simulink model "IEEE123bus_v2019b_Phasor_DPL"  (R2019b)
(part 2 of 7)

  86 : powerlib/Measurements/Three-Phase V-I Measurement  VoltageMeasurement=phase-to-ground  SetLabelV=on  LabelV=V86  Vpu=off  VpuLL=off  CurrentMeasurement=no  SetLabelI=on  LabelI=I65  Ipu=off  Pbase=100e6  Vbase=24900  OutputType=Complex  PhasorSimulation=on  PSBequivalent=0
      settings: SourceProductName=Simscape Electrical
  86 Y PQ : powerlib/Elements/Series RLC Load  LConnTagsString=a  RConnTagsString=__new0  NominalVoltage=1.0*2401.78  NominalFrequency=60  ActivePower=20e3*a  InductivePower=10e3*a  CapacitivePower=0  Setx0=off  InitialVoltage=0  SetiL0=off  InitialCurrent=0  Measurements=None  LoadType=constant PQ
      settings: SourceProductName=Simscape Electrical
  86-87 6 : powerlib/Elements/Distributed Parameters Line  Phases=3  Frequency=60  Resistance=R_3  Inductance=L_3  Capacitance=C_3  Length=450*ft2km  x1=[389.725132711134 3943.58441849278 4019.51592014074;376.991118430775 376.991118430775 376.991118430775;-0.630315628678231 0.166490215186273 1.73524344028808]  x2=[385.27258123151 3942.93848605317 4018.29081213384;376.991118430775 376.991118430775 376.991118430775;-0.627315579650631 0.165297691929816 1.73478902283365]  x3=[26.3237616446647 61.837520404268 25.7980203244257;376.991118430775 376.991118430775 376.991118430775;1.04881280773098 -2.64926297577553 -1.54351880159372]  x4=[26.4518860227079 84.1852813616711 55.6703006140533;376.991118430775 376.991118430775 376.991118430775;-2.0544828369136 0.403647758672959 1.6716643848458]  x5=5.64367487766549e-07  V1=ones(3,3)  V2=ones(3,3)  I1=ones(3,3)  I2=ones(3,3)  nHarmo=1  Measurements=None
      settings: SourceProductName=Simscape Electrical
  87 : powerlib/Measurements/Three-Phase V-I Measurement  VoltageMeasurement=phase-to-ground  SetLabelV=on  LabelV=V87  Vpu=off  VpuLL=off  CurrentMeasurement=no  SetLabelI=on  LabelI=I65  Ipu=off  Pbase=100e6  Vbase=24900  OutputType=Complex  PhasorSimulation=on  PSBequivalent=0
      settings: SourceProductName=Simscape Electrical
  87 Y PQ : powerlib/Elements/Series RLC Load  LConnTagsString=a  RConnTagsString=__new0  NominalVoltage=1.0*2401.78  NominalFrequency=60  ActivePower=40e3*a  InductivePower=20e3*a  CapacitivePower=0  Setx0=off  InitialVoltage=0  SetiL0=off  InitialCurrent=0  Measurements=None  LoadType=constant PQ
      settings: SourceProductName=Simscape Electrical
  87-88 9 : powerlib/Elements/Distributed Parameters Line  Phases=1  Frequency=60  Resistance=R_9(1,1)  Inductance=L_9(1,1)  Capacitance=C_9(1,1)  Length=175*ft2km  x1=[3189.12819557569;376.991118430775;-0.0626467800105766]  x2=[3188.89426292015;376.991118430775;-0.0631855473787039]  x3=[23.2310577601908;376.991118430775;-2.40995823657783]  x4=[32.500362854591;376.991118430775;0.472298354133792]  x5=2.16957196133287e-07  V1=[2.049e+04;377;-2.115]  V2=[2.048e+04;377;-2.115]  I1=[33.62;377;-2.106]  I2=[35.2;377;-2.126]  nHarmo=1  Measurements=None
      settings: SourceProductName=Simscape Electrical
  87-89 6 : powerlib/Elements/Distributed Parameters Line  Phases=3  Frequency=60  Resistance=R_6  Inductance=L_6  Capacitance=C_6  Length=250*ft2km  x1=[473.81611854328 3991.60174475816 3969.04087948509;376.991118430775 376.991118430775 376.991118430775;-1.85006566590342 2.34173752583366 -2.35279833627124]  x2=[472.23324298853 3991.20988754217 3968.71775644618;376.991118430775 376.991118430775 376.991118430775;-1.85482220141547 2.34147098099026 -2.35309575663776]  x3=[27.7854774549557 23.161378351825 22.3415472849966;376.991118430775 376.991118430775 376.991118430775;1.05239756288922 -0.551448243704896 1.00888715490497]  x4=[28.995724845591 52.5570725677784 45.4612866983449;376.991118430775 376.991118430775 376.991118430775;-2.07913897548404 2.45019475060024 -2.24540211987977]  x5=3.13537493203638e-07  V1=ones(3,3)  V2=ones(3,3)  I1=ones(3,3)  I2=ones(3,3)  nHarmo=1  Measurements=None
      settings: SourceProductName=Simscape Electrical
  88 : Subsystem
  88 Y CAP : powerlib/Elements/Series RLC Load  LConnTagsString=a  RConnTagsString=__new0  NominalVoltage=1.0*2401.78  NominalFrequency=60  ActivePower=0  InductivePower=0  CapacitivePower=50e3*a  Setx0=off  InitialVoltage=0  SetiL0=off  InitialCurrent=0  Measurements=None  LoadType=constant PQ
      settings: SourceProductName=Simscape Electrical
  88 Y PQ : powerlib/Elements/Series RLC Load  LConnTagsString=a  RConnTagsString=__new0  NominalVoltage=1.0*2401.78  NominalFrequency=60  ActivePower=40e3*a  InductivePower=20e3*a  CapacitivePower=0  Setx0=off  InitialVoltage=0  SetiL0=off  InitialCurrent=0  Measurements=None  LoadType=constant PQ
      settings: SourceProductName=Simscape Electrical
  89 : powerlib/Measurements/Three-Phase V-I Measurement  VoltageMeasurement=phase-to-ground  SetLabelV=on  LabelV=V89  Vpu=off  VpuLL=off  CurrentMeasurement=no  SetLabelI=on  LabelI=I65  Ipu=off  Pbase=100e6  Vbase=24900  OutputType=Complex  PhasorSimulation=on  PSBequivalent=0
      settings: SourceProductName=Simscape Electrical
  89-90 10 : powerlib/Elements/Distributed Parameters Line  Phases=1  Frequency=60  Resistance=R_10(2,2)  Inductance=L_10(2,2)  Capacitance=C_10(2,2)  Length=225*ft2km  x1=[3294.5580797562;376.991118430775;-2.14263246897096]  x2=[3294.24720092488;376.991118430775;-2.14332515655228]  x3=[23.997649803516;376.991118430775;1.79306719350942]  x4=[33.5736751194491;376.991118430775;-1.60784072680115]  x5=2.78944966457084e-07  V1=[2.049e+04;377;-2.115]  V2=[2.048e+04;377;-2.115]  I1=[33.62;377;-2.106]  I2=[35.2;377;-2.126]  nHarmo=1  Measurements=None
      settings: SourceProductName=Simscape Electrical
  89-91 6 : powerlib/Elements/Distributed Parameters Line  Phases=3  Frequency=60  Resistance=R_6  Inductance=L_6  Capacitance=C_6  Length=225*ft2km  x1=[472.23324298853 3991.20988754217 3968.71775644618;376.991118430775 376.991118430775 376.991118430775;-1.85481038133044 2.34148078793823 -2.35308599234609]  x2=[470.852866317577 3990.95748931504 3968.13044484835;376.991118430775 376.991118430775 376.991118430775;-1.85599036706153 2.34125049686061 -2.35319550645745]  x3=[16.6430406112015 21.0974496754263 13.6262780675171;376.991118430775 376.991118430775 376.991118430775;0.453155732808229 -0.397875664427314 -0.175602388857837]  x4=[17.5009103850392 49.8966502995452 33.1136250740517;376.991118430775 376.991118430775 376.991118430775;-2.63600387714112 2.50767517176072 -2.69801990798261]  x5=2.82183743883275e-07  V1=ones(3,3)  V2=ones(3,3)  I1=ones(3,3)  I2=ones(3,3)  nHarmo=1  Measurements=None
      settings: SourceProductName=Simscape Electrical
  9 : Subsystem
  9 Y PQ : powerlib/Elements/Series RLC Load  LConnTagsString=a  RConnTagsString=__new0  NominalVoltage=1.0*2401.78  NominalFrequency=60  ActivePower=40e3*a  InductivePower=20e3*a  CapacitivePower=0  Setx0=off  InitialVoltage=0  SetiL0=off  InitialCurrent=0  Measurements=None  LoadType=constant PQ
      settings: SourceProductName=Simscape Electrical
  9-14 9 : powerlib/Elements/Distributed Parameters Line  Phases=1  Frequency=60  Resistance=R_9(1,1)  Inductance=L_9(1,1)  Capacitance=C_9(1,1)  Length=425*ft2km  x1=[3293.2882092088;376.991118430775;-0.0226416633012356]  x2=[3287.77688665914;376.991118430775;-0.0232119941323024]  x3=[32.9294633917187;376.991118430775;2.57254896685791]  x4=[43.6783568996041;376.991118430775;-0.425282167284816]  x5=5.26896047752269e-07  V1=[2.049e+04;377;-2.115]  V2=[2.048e+04;377;-2.115]  I1=[33.62;377;-2.106]  I2=[35.2;377;-2.126]  nHarmo=1  Measurements=None
      settings: SourceProductName=Simscape Electrical
  90 : Subsystem
  90 Y CAP : powerlib/Elements/Series RLC Load  LConnTagsString=a  RConnTagsString=__new0  NominalVoltage=1.0*2401.78  NominalFrequency=60  ActivePower=0  InductivePower=0  CapacitivePower=50e3*a  Setx0=off  InitialVoltage=0  SetiL0=off  InitialCurrent=0  Measurements=None  LoadType=constant PQ
      settings: SourceProductName=Simscape Electrical
  90 Y I : powerlib/Elements/Series RLC Load  LConnTagsString=a  RConnTagsString=__new0  NominalVoltage=1.0*2401.78  NominalFrequency=60  ActivePower=40e3*a  InductivePower=20e3*a  CapacitivePower=0  Setx0=off  InitialVoltage=0  SetiL0=off  InitialCurrent=0  Measurements=None  LoadType=constant I
      settings: SourceProductName=Simscape Electrical
  91 : powerlib/Measurements/Three-Phase V-I Measurement  VoltageMeasurement=phase-to-ground  SetLabelV=on  LabelV=V91  Vpu=off  VpuLL=off  CurrentMeasurement=no  SetLabelI=on  LabelI=I65  Ipu=off  Pbase=100e6  Vbase=24900  OutputType=Complex  PhasorSimulation=on  PSBequivalent=0
      settings: SourceProductName=Simscape Electrical
  91-92 11 : powerlib/Elements/Distributed Parameters Line  Phases=1  Frequency=60  Resistance=R_11(3,3)  Inductance=L_11(3,3)  Capacitance=C_11(3,3)  Length=300*ft2km  x1=[3271.58783738673;376.991118430775;2.04939911565278]  x2=[3271.17589452567;376.991118430775;2.04847555887594]  x3=[23.828237165611;376.991118430775;-0.298347801231626]  x4=[33.3379205317264;376.991118430775;2.58396078086368]  x5=3.71926621942778e-07  V1=[2.049e+04;377;-2.115]  V2=[2.048e+04;377;-2.115]  I1=[33.62;377;-2.106]  I2=[35.2;377;-2.126]  nHarmo=1  Measurements=None
      settings: SourceProductName=Simscape Electrical
  91-93 6 : powerlib/Elements/Distributed Parameters Line  Phases=3  Frequency=60  Resistance=R_6  Inductance=L_6  Capacitance=C_6  Length=225*ft2km  x1=[470.852866317578 3990.95748931504 3968.13044484835;376.991118430775 376.991118430775 376.991118430775;-1.85599036706153 2.34125049686061 -2.35319550645745]  x2=[470.681706474968 3990.8003758796 3967.27075184558;376.991118430775 376.991118430775 376.991118430775;-1.85873215043412 2.34117435236502 -2.35329961885097]  x3=[14.3315476659486 2.26149391070465 21.8308711959449;376.991118430775 376.991118430775 376.991118430775;1.54453251115039 2.18854542713267 -0.279792791294667]  x4=[15.530633171256 27.560941394843 38.9320415252189;376.991118430775 376.991118430775 376.991118430775;-1.6175737338596 2.35364341774446 -2.86695357175605]  x5=2.82183743883275e-07  V1=ones(3,3)  V2=ones(3,3)  I1=ones(3,3)  I2=ones(3,3)  nHarmo=1  Measurements=None
      settings: SourceProductName=Simscape Electrical
  92 : Subsystem
  92 Y CAP : powerlib/Elements/Series RLC Load  LConnTagsString=a  RConnTagsString=__new0  NominalVoltage=1.0*2401.78  NominalFrequency=60  ActivePower=0  InductivePower=0  CapacitivePower=50e3*a  Setx0=off  InitialVoltage=0  SetiL0=off  InitialCurrent=0  Measurements=None  LoadType=constant PQ
      settings: SourceProductName=Simscape Electrical
  92 Y PQ : powerlib/Elements/Series RLC Load  LConnTagsString=a  RConnTagsString=__new0  NominalVoltage=1.0*2401.78  NominalFrequency=60  ActivePower=40e3*a  InductivePower=20e3*a  CapacitivePower=0  Setx0=off  InitialVoltage=0  SetiL0=off  InitialCurrent=0  Measurements=None  LoadType=constant PQ
      settings: SourceProductName=Simscape Electrical
  93 : powerlib/Measurements/Three-Phase V-I Measurement  VoltageMeasurement=phase-to-ground  SetLabelV=on  LabelV=V93  Vpu=off  VpuLL=off  CurrentMeasurement=no  SetLabelI=on  LabelI=I65  Ipu=off  Pbase=100e6  Vbase=24900  OutputType=Complex  PhasorSimulation=on  PSBequivalent=0
      settings: SourceProductName=Simscape Electrical
  93-94 9 : powerlib/Elements/Distributed Parameters Line  Phases=1  Frequency=60  Resistance=R_9(1,1)  Inductance=L_9(1,1)  Capacitance=C_9(1,1)  Length=275*ft2km  x1=[3186.20288003371;376.991118430775;-0.0626781017533015]  x2=[3183.89965413122;376.991118430775;-0.0629245614320662]  x3=[19.6379798328121;376.991118430775;2.48172169950306]  x4=[30.0102267929362;376.991118430775;-0.439582531686713]  x5=3.4093273678088e-07  V1=[2.049e+04;377;-2.115]  V2=[2.048e+04;377;-2.115]  I1=[33.62;377;-2.106]  I2=[35.2;377;-2.126]  nHarmo=1  Measurements=None
      settings: SourceProductName=Simscape Electrical
  93-95 6 : powerlib/Elements/Distributed Parameters Line  Phases=3  Frequency=60  Resistance=R_6  Inductance=L_6  Capacitance=C_6  Length=300*ft2km  x1=[470.681706474968 3990.8003758796 3967.27075184558;376.991118430775 376.991118430775 376.991118430775;-1.85876761068919 2.34114493152109 -2.35332891172598]  x2=[469.094791066072 3990.70610382809 3966.75981157663;376.991118430775 376.991118430775 376.991118430775;-1.86036423757392 2.34116651569893 -2.35349294353194]  x3=[14.6489363119123 16.0990590981964 8.28991857832063;376.991118430775 376.991118430775 376.991118430775;0.505634596158928 2.55692710302294 0.172441929984786]  x4=[15.5543418042633 14.4835044327244 30.5310486561755;376.991118430775 376.991118430775 376.991118430775;-2.58028850236118 2.10074268853675 -2.51092860023359]  x5=3.76244991844366e-07  V1=ones(3,3)  V2=ones(3,3)  I1=ones(3,3)  I2=ones(3,3)  nHarmo=1  Measurements=None
      settings: SourceProductName=Simscape Electrical
  94 : Subsystem
  94 Y PQ : powerlib/Elements/Series RLC Load  LConnTagsString=a  RConnTagsString=__new0  NominalVoltage=1.0*2401.78  NominalFrequency=60  ActivePower=40e3*a  InductivePower=20e3*a  CapacitivePower=0  Setx0=off  InitialVoltage=0  SetiL0=off  InitialCurrent=0  Measurements=None  LoadType=constant PQ
      settings: SourceProductName=Simscape Electrical
  95 : powerlib/Measurements/Three-Phase V-I Measurement  VoltageMeasurement=phase-to-ground  SetLabelV=on  LabelV=V95  Vpu=off  VpuLL=off  CurrentMeasurement=no  SetLabelI=on  LabelI=I65  Ipu=off  Pbase=100e6  Vbase=24900  OutputType=Complex  PhasorSimulation=on  PSBequivalent=0
      settings: SourceProductName=Simscape Electrical
  95 Y PQ : powerlib/Elements/Series RLC Load  LConnTagsString=a  RConnTagsString=__new0  NominalVoltage=1.0*2401.78  NominalFrequency=60  ActivePower=20e3*a  InductivePower=10e3*a  CapacitivePower=0  Setx0=off  InitialVoltage=0  SetiL0=off  InitialCurrent=0  Measurements=None  LoadType=constant PQ
      settings: SourceProductName=Simscape Electrical
  95-96 10 : powerlib/Elements/Distributed Parameters Line  Phases=1  Frequency=60  Resistance=R_10(2,2)  Inductance=L_10(2,2)  Capacitance=C_10(2,2)  Length=200*ft2km  x1=[3291.68223176676;376.991118430775;-2.14349881403869]  x2=[3290.81659855226;376.991118430775;-2.1435884793496]  x3=[7.8420771963233;376.991118430775;0.183451795456017]  x4=[18.3446926798263;376.991118430775;-2.45979310961386]  x5=2.47951081295186e-07  V1=[2.049e+04;377;-2.115]  V2=[2.048e+04;377;-2.115]  I1=[33.62;377;-2.106]  I2=[35.2;377;-2.126]  nHarmo=1  Measurements=None
      settings: SourceProductName=Simscape Electrical
  96 : Subsystem
  96 Y PQ : powerlib/Elements/Series RLC Load  LConnTagsString=a  RConnTagsString=__new0  NominalVoltage=1.0*2401.78  NominalFrequency=60  ActivePower=20e3*a  InductivePower=10e3*a  CapacitivePower=0  Setx0=off  InitialVoltage=0  SetiL0=off  InitialCurrent=0  Measurements=None  LoadType=constant PQ
      settings: SourceProductName=Simscape Electrical
  97 : powerlib/Measurements/Three-Phase V-I Measurement  VoltageMeasurement=phase-to-ground  SetLabelV=on  LabelV=V97  Vpu=off  VpuLL=off  CurrentMeasurement=no  SetLabelI=on  LabelI=I65  Ipu=off  Pbase=100e6  Vbase=24900  OutputType=Complex  PhasorSimulation=on  PSBequivalent=0
      settings: SourceProductName=Simscape Electrical
  97-1 : powerlib/Elements/Three-Phase Breaker  InitialState=closed  SwitchA=off  SwitchB=off  SwitchC=off  SwitchTimes="[1/60  5/60]"  External=off  BreakerResistance=0.01  SnubberResistance=1e6  SnubberCapacitance=inf  Measurements=None
      settings: SourceProductName=Simscape Electrical
  97-98 3 : powerlib/Elements/Distributed Parameters Line  Phases=3  Frequency=60  Resistance=R_3  Inductance=L_3  Capacitance=C_3  Length=275*ft2km  x1=[403.937531783188 3940.87502820857 4020.59041973766;376.991118430775 376.991118430775 376.991118430775;-0.646391019388133 0.171790040209764 1.73773895557919]  x2=[403.861142613594 3939.94266678301 4019.74449789447;376.991118430775 376.991118430775 376.991118430775;-0.646346774908461 0.171591937014733 1.7375941915319]  x3=[0.839908291662697 20.8341181628027 18.9160993242188;376.991118430775 376.991118430775 376.991118430775;0.401209150214837 2.60032529534016 -2.23068888651644]  x4=[0.970391891284456 41.3016543620584 45.0288249680596;376.991118430775 376.991118430775 376.991118430775;-1.49414554390316 -0.164580907224629 1.42340618711029]  x5=3.44891242524002e-07  V1=ones(3,3)  V2=ones(3,3)  I1=ones(3,3)  I2=ones(3,3)  nHarmo=1  Measurements=None
      settings: SourceProductName=Simscape Electrical
  98 : powerlib/Measurements/Three-Phase V-I Measurement  VoltageMeasurement=phase-to-ground  SetLabelV=on  LabelV=V98  Vpu=off  VpuLL=off  CurrentMeasurement=no  SetLabelI=on  LabelI=I65  Ipu=off  Pbase=100e6  Vbase=24900  OutputType=Complex  PhasorSimulation=on  PSBequivalent=0
      settings: SourceProductName=Simscape Electrical
  98 Y PQ : powerlib/Elements/Series RLC Load  LConnTagsString=a  RConnTagsString=__new0  NominalVoltage=1.0*2401.78  NominalFrequency=60  ActivePower=40e3*a  InductivePower=20e3*a  CapacitivePower=0  Setx0=off  InitialVoltage=0  SetiL0=off  InitialCurrent=0  Measurements=None  LoadType=constant PQ
      settings: SourceProductName=Simscape Electrical
  98-99 3 : powerlib/Elements/Distributed Parameters Line  Phases=3  Frequency=60  Resistance=R_3  Inductance=L_3  Capacitance=C_3  Length=550*ft2km  x1=[403.861142613594 3939.94266678301 4019.74449789447;376.991118430775 376.991118430775 376.991118430775;-0.646476795843717 0.17148452980637 1.73748631510416]  x2=[404.519233586383 3939.39361708882 4017.96938193094;376.991118430775 376.991118430775 376.991118430775;-0.638932394717352 0.171255069019233 1.73724918128971]  x3=[15.1568739438104 2.36811354238008 19.6804091305056;376.991118430775 376.991118430775 376.991118430775;-0.47975750385127 2.46520645653906 -2.40465479538252]  x4=[14.1095696620574 24.8542542995005 43.8760242147607;376.991118430775 376.991118430775 376.991118430775;2.67406062113987 0.0997675642856184 1.35014718321215]  x5=6.89782485048005e-07  V1=ones(3,3)  V2=ones(3,3)  I1=ones(3,3)  I2=ones(3,3)  nHarmo=1  Measurements=None
      settings: SourceProductName=Simscape Electrical
  99 : powerlib/Measurements/Three-Phase V-I Measurement  VoltageMeasurement=phase-to-ground  SetLabelV=on  LabelV=V99  Vpu=off  VpuLL=off  CurrentMeasurement=no  SetLabelI=on  LabelI=I65  Ipu=off  Pbase=100e6  Vbase=24900  OutputType=Complex  PhasorSimulation=on  PSBequivalent=0
      settings: SourceProductName=Simscape Electrical
  99 Y PQ : powerlib/Elements/Series RLC Load  LConnTagsString=a  RConnTagsString=__new0  NominalVoltage=1.0*2401.78  NominalFrequency=60  ActivePower=40e3*a  InductivePower=20e3*a  CapacitivePower=0  Setx0=off  InitialVoltage=0  SetiL0=off  InitialCurrent=0  Measurements=None  LoadType=constant PQ
      settings: SourceProductName=Simscape Electrical
  99-100 3 : powerlib/Elements/Distributed Parameters Line  Phases=3  Frequency=60  Resistance=R_3  Inductance=L_3  Capacitance=C_3  Length=300*ft2km  x1=[404.519233586383 3939.39361708882 4017.96938193094;376.991118430775 376.991118430775 376.991118430775;-0.638814193867119 0.171352711935926 1.73734725076947]  x2=[406.131749441997 3939.12031039649 4017.5206124443;376.991118430775 376.991118430775 376.991118430775;-0.637696739708932 0.171396814501649 1.73720135136297]  x3=[14.7350627090076 14.7374367546136 6.09153248747518;376.991118430775 376.991118430775 376.991118430775;-1.52510205388982 0.695519460331209 -1.92780172841348]  x4=[14.0859959320792 12.8021670637714 35.4013446196294;376.991118430775 376.991118430775 376.991118430775;1.55783195926751 -0.442738598732068 1.6510997033146]  x5=3.76244991844366e-07  V1=ones(3,3)  V2=ones(3,3)  I1=ones(3,3)  I2=ones(3,3)  nHarmo=1  Measurements=None
      settings: SourceProductName=Simscape Electrical
  Ground{,1..81} (82 alike) : powerlib/Elements/Ground  LConnTagsString=a
      settings: SourceProductName=Simscape Electrical
  Load Flow Bus10 : powerlib/Measurements/Load Flow Bus  LConnTagsString=a|b|c  Phases=ABC  Connectors=on one side  ID=251  Vbase=4160/sqrt(3)  Vref=[1.0 1.0 1.0]  Vangle=[0 -120 120]  VLF=1  VLFb=1  VLFc=1  angleLF=0  angleLFb=0  angleLFc=0
      settings: SourceProductName=Simscape Electrical
  Load Flow Bus106 : powerlib/Measurements/Load Flow Bus  LConnTagsString=a|b|c  RConnTagsString=a|b|c  Phases=ABC  Connectors=on both sides  ID=450  Vbase=4160/sqrt(3)  Vref=[1.0 1.0 1.0]  Vangle=[0 -120 120]  VLF=1  VLFb=1  VLFc=1  angleLF=0  angleLFb=0  angleLFc=0
      settings: SourceProductName=Simscape Electrical
  Load Flow Bus107 : powerlib/Measurements/Load Flow Bus  LConnTagsString=a|b|c  Phases=ABC  Connectors=on one side  ID=451  Vbase=4160/sqrt(3)  Vref=[1.0 1.0 1.0]  Vangle=[0 -120 120]  VLF=1  VLFb=1  VLFc=1  angleLF=0  angleLFb=0  angleLFc=0
      settings: SourceProductName=Simscape Electrical
  Load Flow Bus117 : powerlib/Measurements/Load Flow Bus  LConnTagsString=a|b|c  Phases=ABC  Connectors=on one side  ID=79  Vbase=4160/sqrt(3)  Vref=[1.0 1.0 1.0]  Vangle=[0 -120 120]  VLF=1  VLFb=1  VLFc=1  angleLF=0  angleLFb=0  angleLFc=0
      settings: SourceProductName=Simscape Electrical
  Load Flow Bus128 : powerlib/Measurements/Load Flow Bus  LConnTagsString=a|b|c  Phases=ABC  Connectors=on one side  ID=66  Vbase=4160/sqrt(3)  Vref=[1.0 1.0 1.0]  Vangle=[0 -120 120]  VLF=1  VLFb=1  VLFc=1  angleLF=0  angleLFb=0  angleLFc=0
      settings: SourceProductName=Simscape Electrical
  Load Flow Bus2 : powerlib/Measurements/Load Flow Bus  LConnTagsString=a|b|c  RConnTagsString=a|b|c  Phases=ABC  Connectors=on both sides  ID=36  Vbase=4160/sqrt(3)  Vref=[1.0 1.0]  Vangle=[0 -120]  VLF=1  VLFb=1  VLFc=1  angleLF=0  angleLFb=0  angleLFc=0
      settings: SourceProductName=Simscape Electrical
  Load Flow Bus44 : powerlib/Measurements/Load Flow Bus  LConnTagsString=a|b|c  RConnTagsString=a|b|c  Phases=ABC  Connectors=on both sides  ID=300  Vbase=4160/sqrt(3)  Vref=[1.0 1.0 1.0]  Vangle=[0 -120 120]  VLF=1  VLFb=1  VLFc=1  angleLF=0  angleLFb=0  angleLFc=0
      settings: SourceProductName=Simscape Electrical
  Load Flow Bus45 : powerlib/Measurements/Load Flow Bus  LConnTagsString=a|b|c  Phases=ABC  Connectors=on one side  ID=350  Vbase=4160/sqrt(3)  Vref=[1.0 1.0 1.0]  Vangle=[0 -120 120]  VLF=1  VLFb=1  VLFc=1  angleLF=0  angleLFb=0  angleLFc=0
      settings: SourceProductName=Simscape Electrical
  Load Flow Bus55 : powerlib/Measurements/Load Flow Bus  LConnTagsString=a|b  RConnTagsString=a|b  Phases=AB  Connectors=on both sides  ID=36  Vbase=4160/sqrt(3)  Vref=[1.0 1.0]  Vangle=[0 -120]  VLF=1  VLFb=1  VLFc=1  angleLF=0  angleLFb=0  angleLFc=0
      settings: SourceProductName=Simscape Electrical
  Load Flow Bus68 : powerlib/Measurements/Load Flow Bus  LConnTagsString=a|b|c  Phases=ABC  Connectors=on one side  ID=56  Vbase=4160/sqrt(3)  Vref=[1.0 1.0 1.0]  Vangle=[0 -120 120]  VLF=1  VLFb=1  VLFc=1  angleLF=0  angleLFb=0  angleLFc=0
      settings: SourceProductName=Simscape Electrical
  Load Flow Bus77 : powerlib/Measurements/Load Flow Bus  LConnTagsString=a|b|c  RConnTagsString=a|b|c  Phases=ABC  Connectors=on both sides  ID=95  Vbase=4160/sqrt(3)  Vref=[1.0 1.0 1.0]  Vangle=[0 -120 120]  VLF=1  VLFb=1  VLFc=1  angleLF=0  angleLFb=0  angleLFc=0
      settings: SourceProductName=Simscape Electrical
  Load Flow Bus78 : powerlib/Measurements/Load Flow Bus  LConnTagsString=a|b|c  Phases=ABC  Connectors=on one side  ID=195  Vbase=4160/sqrt(3)  Vref=[1.0 1.0 1.0]  Vangle=[0 -120 120]  VLF=1  VLFb=1  VLFc=1  angleLF=0  angleLFb=0  angleLFc=0
      settings: SourceProductName=Simscape Electrical
  Load Flow Bus84 : powerlib/Measurements/Load Flow Bus  Commented=on  LConnTagsString=a|b|c  Phases=ABC  Connectors=on one side  ID=610  Vbase=480/sqrt(3)  Vref=[1.0 1.0 1.0]  Vangle=[0 -120 120]  VLF=1  VLFb=1  VLFc=1  angleLF=0  angleLFb=0  angleLFc=0
      settings: SourceProductName=Simscape Electrical
  Measurements : Subsystem
  RG1in : powerlib/Measurements/Three-Phase V-I Measurement  VoltageMeasurement=phase-to-ground  SetLabelV=on  LabelV=RG1in  Vpu=off  VpuLL=off  CurrentMeasurement=no  SetLabelI=on  LabelI=I800  Ipu=off  Pbase=100e6  Vbase=24900  OutputType=Complex  PhasorSimulation=on  PSBequivalent=0
      settings: SourceProductName=Simscape Electrical
  RG1out : powerlib/Measurements/Three-Phase V-I Measurement  VoltageMeasurement=phase-to-ground  SetLabelV=on  LabelV=RG1out  Vpu=off  VpuLL=off  CurrentMeasurement=no  SetLabelI=on  LabelI=I800  Ipu=off  Pbase=100e6  Vbase=24900  OutputType=Complex  PhasorSimulation=on  PSBequivalent=0
      settings: SourceProductName=Simscape Electrical
  RG2in : Subsystem
  RG2out : Subsystem
  RG3in : Subsystem
  RG3out : Subsystem
  RG4in : powerlib/Measurements/Three-Phase V-I Measurement  VoltageMeasurement=phase-to-ground  SetLabelV=on  LabelV=RG4in  Vpu=off  VpuLL=off  CurrentMeasurement=no  SetLabelI=on  LabelI=I800  Ipu=off  Pbase=100e6  Vbase=24900  OutputType=Complex  PhasorSimulation=on  PSBequivalent=0
      settings: SourceProductName=Simscape Electrical
  RG4out : powerlib/Measurements/Three-Phase V-I Measurement  VoltageMeasurement=phase-to-ground  SetLabelV=on  LabelV=RG4out  Vpu=off  VpuLL=off  CurrentMeasurement=no  SetLabelI=on  LabelI=I800  Ipu=off  Pbase=100e6  Vbase=24900  OutputType=Complex  PhasorSimulation=on  PSBequivalent=0
      settings: SourceProductName=Simscape Electrical
  Regulator 1 Three Phase Ganged SVR : Subsystem
  Regulator 2 : Subsystem
  Regulator 3 : Subsystem
  Regulator 4 : Subsystem
  Regulator Taps : Subsystem
  Series RLC Branch1 : powerlib/Elements/Series RLC Branch  LConnTagsString=__new0  RConnTagsString=__new0  BranchType=R  Resistance=.001  Inductance=0  SetiL0=off  InitialCurrent=0  Capacitance=0  Setx0=off  InitialVoltage=0  Measurements=None
      settings: SourceProductName=Simscape Electrical
  Series RLC Branch2 : powerlib/Elements/Series RLC Branch  LConnTagsString=__new0  RConnTagsString=__new0  BranchType=R  Resistance=.001  Inductance=0  SetiL0=off  InitialCurrent=0  Capacitance=0  Setx0=off  InitialVoltage=0  Measurements=None
      settings: SourceProductName=Simscape Electrical
  Series RLC Branch3 : powerlib/Elements/Series RLC Branch  LConnTagsString=__new0  RConnTagsString=__new0  BranchType=R  Resistance=.001  Inductance=0  SetiL0=off  InitialCurrent=0  Capacitance=0  Setx0=off  InitialVoltage=0  Measurements=None
      settings: SourceProductName=Simscape Electrical
  Substation Power : Subsystem
  Three-Phase Transformer (Two Windings) : powerlib/Elements/Three-Phase Transformer (Two Windings)  Winding1Connection=Delta (D1)  Winding2Connection=Delta (D1)  CoreType=Three single-phase transformers  SetSaturation=off  Hysteresis=off  DataFile='hysteresis'  SetInitialFlux=off  Measurements=None  UNITS=pu  NominalPower=[ 500e3 , 60 ]  Winding1=[4160 0.0127 0.0272]  Winding2=[480 0.0127 0.0272]  Rm=1000  Lm=1000  L0=0.5  Saturation=[ 0,0 ; 0.0024,1.2 ; 1.0,1.52 ]  InitialFluxes=[ 0.8 , -0.8 , 0.7 ]  BreakLoop=on  DiscreteSolver=Trapezoidal iterative  DataType=off  TransfoNumber=1
      settings: SourceProductName=Simscape Electrical
  Three-Phase Breaker1 : powerlib/Elements/Three-Phase Breaker  InitialState=open  SwitchA=off  SwitchB=off  SwitchC=off  SwitchTimes="[1/60  5/60]"  External=off  BreakerResistance=0.01  SnubberResistance=1e6  SnubberCapacitance=inf  Measurements=None
      settings: SourceProductName=Simscape Electrical
  XF1 : powerlib/Measurements/Three-Phase V-I Measurement  VoltageMeasurement=phase-to-ground  SetLabelV=on  LabelV=XF1  Vpu=off  VpuLL=off  CurrentMeasurement=no  SetLabelI=on  LabelI=I65  Ipu=off  Pbase=100e6  Vbase=24900  OutputType=Complex  PhasorSimulation=on  PSBequivalent=0
      settings: SourceProductName=Simscape Electrical
  powergui : powerlib/powergui  Priority=1  SimulationMode=Phasor  SampleTime=Ts  frequency=60  Iterations=50  frequencyindice=0  Pbase=100e6  ErrMax=1e-4  UnitsV=kV  UnitsW=MW  buscounter=0  FunctionMessages=off  echomessages=on  EnableUseOfTLC=off  CurrentSourceSwitches=off  DisableSnubberDevices=off  DisableRonSwitches=off  DisableVfSwitches=off  DisplayEquations=off  AutomaticDiscreteSolvers=off  SolverType=Tustin/Backward Euler (TBE)  Interpol=off  ExternalGateDelay=off  methode=off  Ts=0  x0status=blocks  SPID=off  SwTol=0  HookPort=off  NonlinearTolerance=1e-4  nMaxIteration=100  ContinueOnMaxIteration=off  RestoreLinks=warning  ResistiveCurrentMeasurement=off  Frange=[0:2:500]  Ylog=off  Xlog=on  ShowGrid=off  save=off  variable=ZData  structure=0  ZoomFFT=off  StartTime=0.0  cycles=1  DisplayStyle=1  fundamental=60  FreqAxis=off  MaxFrequency=1000  frequencyindicesteady=1  RmsSteady=1  display=off
      settings: SourceProductName=Simscape Electrical
  tag scope: Reg1=global, Reg2=global, Reg3=global, Reg4=global
  wires:
  Regulator 1 Three Phase Ganged SVR/1(Tap) -> [Reg1]
  Regulator 4/1(Tap) -> [Reg4]
  Regulator 2/1(Tap) -> [Reg2]
  Regulator 3/1(Taps) -> [Reg3]
  connections:
  25-26 1/RConn1 -- 26-31 1/LConn1 -- 26/LConn2
  51-151 4/RConn3 -- 151/RConn3
  51-151 4/RConn2 -- 151/RConn2
  51-151 4/RConn1 -- 151/RConn1
  Regulator 1 Three Phase Ganged SVR/RConn3 -- RG1out/LConn3
  Regulator 1 Three Phase Ganged SVR/RConn2 -- RG1out/LConn2
  Regulator 1 Three Phase Ganged SVR/RConn1 -- RG1out/LConn1
  Regulator 1 Three Phase Ganged SVR/LConn3 -- RG1in/RConn3
  Regulator 1 Three Phase Ganged SVR/LConn2 -- RG1in/RConn2
  Regulator 1 Three Phase Ganged SVR/LConn1 -- RG1in/RConn1
  Series RLC Branch2/LConn1 -- 4160 V swing/RConn3
  Series RLC Branch1/LConn1 -- 4160 V swing/RConn2
  Series RLC Branch3/LConn1 -- 4160 V swing/RConn1
  Series RLC Branch2/RConn1 -- 150/LConn3
  Series RLC Branch1/RConn1 -- 150/LConn2
  Series RLC Branch3/RConn1 -- 150/LConn1
  Load Flow Bus2/LConn3 -- 35/RConn3
  Load Flow Bus2/LConn2 -- 35/RConn2
  Load Flow Bus2/LConn1 -- 35/RConn1
  61-610/RConn3 -- XF1/LConn3
  XF1/RConn3 -- Three-Phase Transformer (Two Windings)/LConn3
  RG1out/RConn3 -- 149/LConn3
  RG1out/RConn2 -- 149/LConn2
  RG1out/RConn1 -- 149/LConn1
  RG2out/RConn1 -- 14/LConn1
  160 67 6/RConn3 -- RG4in/LConn3
  160 67 6/RConn2 -- RG4in/LConn2
  160 67 6/RConn1 -- RG4in/LConn1
  9-14 9/RConn1 -- RG2in/LConn1
  610/RConn3 -- Load Flow Bus84/LConn3
  610/RConn2 -- Load Flow Bus84/LConn2
  610/RConn1 -- Load Flow Bus84/LConn1
  610/LConn3 -- Three-Phase Transformer (Two Windings)/RConn3
  610/LConn2 -- Three-Phase Transformer (Two Windings)/RConn2
  610/LConn1 -- Three-Phase Transformer (Two Windings)/RConn1
  XF1/RConn2 -- Three-Phase Transformer (Two Windings)/LConn2
  XF1/RConn1 -- Three-Phase Transformer (Two Windings)/LConn1
  XF1/LConn2 -- 61-610/RConn2
  XF1/LConn1 -- 61-610/RConn1
  85/RConn1 -- 85 Y PQ/LConn1
  75 Y PQ/LConn1 -- 75/RConn1
  71/RConn1 -- 71 Y PQ/LConn1
  103-104 11/RConn1 -- 104/LConn1
  106-107 10/RConn1 -- 107/LConn1
  114/RConn1 -- 114 Y PQ/LConn1
  111/RConn1 -- 111 Y PQ/LConn1
  87-88 9/RConn1 -- 88/LConn1
  89-90 10/RConn1 -- 90/LConn1
  91-92 11/RConn1 -- 92/LConn1
  96 Y PQ/LConn1 -- 96/RConn1
  15-17 11/RConn1 -- 17/LConn1
  15-16 11/RConn1 -- 16/LConn1
  59 Y PQ/LConn1 -- 59/RConn1
  57-58 10/LConn1 -- 58/LConn1
  36/RConn2 -- Load Flow Bus55/LConn2
  36/LConn2 -- 35-36 8/RConn2
  36/RConn1 -- Load Flow Bus55/LConn1
  37 Y Z/LConn1 -- 37/RConn1
  38-39 10/RConn1 -- 39/LConn1
  41/RConn1 -- 41 Y PQ/LConn1
  43/RConn1 -- 43 Y Z/LConn1
  45-46 9/RConn1 -- 46/LConn1
  31-32 1/RConn1 -- 32/LConn1
  33 Y I/LConn1 -- 33/RConn1
  27-33 1/LConn1 -- 27/RConn1
  23-24 11/RConn1 -- 24/LConn1
  21-22 10/RConn1 -- 22/LConn1
  20/RConn1 -- 20 Y I/LConn1
  95/RConn3 -- Load Flow Bus77/RConn3
  95/RConn2 -- Load Flow Bus77/RConn2
  95/RConn1 -- Load Flow Bus77/RConn1
  79/RConn3 -- Load Flow Bus117/LConn3
  79/RConn2 -- Load Flow Bus117/LConn2
  78-79 6/RConn3 -- 79/LConn3
  78-79 6/RConn2 -- 79/LConn2
  78-79 6/RConn1 -- 79/LConn1
  151/LConn3 -- 151-1/LConn3
  151/LConn2 -- 151-1/LConn2
  151/LConn1 -- 151-1/LConn1
  300/RConn3 -- Load Flow Bus44/LConn3
  300/RConn2 -- Load Flow Bus44/LConn2
  300/RConn1 -- Load Flow Bus44/LConn1
  450/RConn3 -- Load Flow Bus106/LConn3
  450/RConn2 -- Load Flow Bus106/LConn2
  450/RConn1 -- Load Flow Bus106/LConn1
  100-450 3/RConn3 -- 450/LConn3
  100-450 3/RConn2 -- 450/LConn2
  100-450 3/RConn1 -- 450/LConn1
  56/RConn3 -- Load Flow Bus68/LConn3
  56/RConn1 -- Load Flow Bus68/LConn1
  55-56 1/RConn3 -- 56/LConn3
  55-56 1/RConn2 -- 56/LConn2
  55-56 1/RConn1 -- 56/LConn1
  66/RConn2 -- Load Flow Bus128/LConn2
  66/RConn1 -- Load Flow Bus128/LConn1
  65-66 12/RConn3 -- 66/LConn3
  65-66 12/RConn2 -- 66/LConn2
  65-66 12/RConn1 -- 66/LConn1
  51-151 4/LConn3 -- 51/RConn3
  51-151 4/LConn2 -- 51/RConn2
  50-51 4/RConn3 -- 51/LConn3
  50-51 4/RConn2 -- 51/LConn2
  50-51 4/RConn1 -- 51/LConn1
  48/LConn3 -- 48 Y Z/LConn3
  48 Y Z/LConn2 -- 48/LConn2
  48/LConn1 -- 48 Y Z/LConn1
  8-12 10/RConn1 -- 12/LConn1
  6/RConn1 -- 6 Y Z/LConn1
  4Y PQ/LConn1 -- 4/RConn1
  11/RConn1 -- 11 Y Z/LConn1
  14-10 9/LConn1 -- 10/LConn1
  1-2 10/RConn1 -- 2/LConn1
  RG1in/LConn3 -- 150-1/RConn3
  RG1in/LConn2 -- 150-1/RConn2
  RG1in/LConn1 -- 150-1/RConn1
  1/RConn3 -- 1-3 11/LConn1 -- 1-7 1/LConn3
  1-7 1/LConn2 -- 1/RConn2
  1 Y PQ/LConn1 -- 1-7 1/LConn1 -- 1/RConn1
  Load Flow Bus44/RConn2 -- 300-1/LConn2
  Load Flow Bus44/RConn1 -- 300-1/LConn1
  300-1/RConn3 -- Load Flow Bus45/LConn3
  300-1/RConn2 -- Load Flow Bus45/LConn2
  300-1/RConn1 -- Load Flow Bus45/LConn1
  197/LConn3 -- 97-1/RConn3
  197/LConn2 -- 97-1/RConn2
  197/LConn1 -- 97-1/RConn1
  18-135/LConn3 -- 18-21 2/LConn3 -- 18/RConn3
  18-135/LConn2 -- 18-21 2/LConn2 -- 18/RConn2
  18-21 2/LConn1 -- 18-19 9/LConn1 -- 18-135/LConn1 -- 18/RConn1
  150/RConn3 -- 150-1/LConn3
  150/RConn1 -- 150-1/LConn1
  61/RConn3 -- 61-610/LConn3
  61/RConn2 -- 61-610/LConn2
  61/RConn1 -- 61-610/LConn1
  160 67 6/LConn1 -- 160/RConn1
  160 67 6/LConn2 -- 160/RConn2
  54/LConn1 -- 54-57 3/LConn1 -- 53-54 1/RConn1 -- 59-94/LConn1
  Three-Phase Breaker1/LConn3 -- 93-95 6/RConn3 -- 95/LConn3
  Three-Phase Breaker1/LConn2 -- 93-95 6/RConn2 -- 95/LConn2 -- 95 Y PQ/LConn1
  Three-Phase Breaker1/LConn1 -- 93-95 6/RConn1 -- 95/LConn1
  450-451/LConn3 -- Load Flow Bus106/RConn3
  Load Flow Bus106/RConn2 -- 450-451/LConn2
  Load Flow Bus106/RConn1 -- 450-451/LConn1
  Load Flow Bus44/RConn3 -- 300-1/LConn3
  250/RConn3 -- 250-251/LConn3
  250/RConn2 -- 250-251/LConn2
  250/RConn1 -- 250-251/LConn1
  135/LConn3 -- 18-135/RConn3
  135/LConn2 -- 18-135/RConn2
  135/LConn1 -- 18-135/RConn1
  35-40 1/RConn2 -- 40/LConn2
  35-40 1/RConn1 -- 40/LConn1
  35-40 1/RConn3 -- 40/LConn3
  77-78 6/LConn3 -- 77/RConn3
  77-78 6/LConn1 -- 77/RConn1
  77-78 6/LConn2 -- 77/RConn2
  87-89 6/LConn3 -- 87/RConn3
  87 Y PQ/LConn1 -- 87-89 6/LConn2 -- 87/RConn2
  34-15 11/RConn1 -- 15/LConn1
  64-65 12/LConn3 -- 64/RConn3
  64-65 12/LConn2 -- 64/RConn2
  64-65 12/LConn1 -- 64/RConn1
  110-112 9/LConn1 -- 110/RConn1
  54-55 1/RConn3 -- 55/LConn3
  54-55 1/RConn1 -- 55/LConn1
  54-55 1/RConn2 -- 55/LConn2
  74 Y Z/LConn1 -- 73-74 11/RConn1 -- 74/LConn1
  50-51 4/LConn3 -- 50/RConn3
  50-51 4/LConn2 -- 50/RConn2
  50-51 4/LConn1 -- 50/RConn1
  30-250 2/LConn3 -- "30 "/RConn3
  30-250 2/LConn2 -- "30 "/RConn2
  30-250 2/LConn1 -- "30 "/RConn1
  98-99 3/LConn3 -- 98/RConn3
  98-99 3/LConn2 -- 98/RConn2
  98 Y PQ/LConn1 -- 98-99 3/LConn1 -- 98/RConn1
  57-60 3/LConn1 -- 57/LConn1
  57-60 3/LConn3 -- 57/LConn3
  57-60 3/LConn2 -- 57/LConn2
  7-8 1/LConn3 -- 7/RConn3
  7-8 1/LConn2 -- 7/RConn2
  7-8 1/LConn1 -- 7/RConn1
  91-93 6/RConn1 -- 93/LConn1
  91-93 6/RConn3 -- 93/LConn3
  91-93 6/RConn2 -- 93/LConn2
  81-82 6/LConn2 -- 81/RConn2
  81-82 6/LConn1 -- 81/RConn1
  72-76 3/LConn3 -- 72/RConn3
  72-76 3/LConn2 -- 72/RConn2
  72-76 3/LConn1 -- 72/RConn1
  101-105 3/LConn3 -- 101/RConn3
  101-105 3/LConn2 -- 101/RConn2
  101-105 3/LConn1 -- 101/RConn1
  108-300 3/LConn3 -- 108/RConn3
  108-300 3/LConn2 -- 108/RConn2
  108/RConn1 -- 108-300 3/LConn1 -- 108-109 9/LConn1
  44-47 1/LConn3 -- 44/RConn3
  44-47 1/LConn2 -- 44/RConn2
  25-28 2/LConn3 -- 25/RConn3
  25-28 2/LConn2 -- 25/RConn2
  25-28 2/LConn1 -- 25/RConn1
  160 67 6/LConn3 -- 160/RConn3
  13-152/RConn3 -- 152/LConn3
  13-152/RConn2 -- 152/LConn2
  13-152/RConn1 -- 152/LConn1
  65 D Z/LConn1 -- 64-65 12/RConn1 -- 65/LConn1
  65 D Z/LConn3 -- 64-65 12/RConn3 -- 65/LConn3
  55 Y Z/LConn1 -- 55-56 1/LConn1 -- 55/RConn1
  55-56 1/LConn2 -- 55/RConn2
  55-56 1/LConn3 -- 55/RConn3
  51 Y PQ/LConn1 -- 51-151 4/LConn1 -- 51/RConn1
  21-23 2/LConn1 -- 21/RConn1
  27-33 1/RConn1 -- 33/LConn1
  67-72 3/RConn3 -- 72/LConn3
  56 Y PQ/LConn1 -- Load Flow Bus68/LConn2 -- 56/RConn2
  25/LConn3 -- 23-25 2/RConn3 -- RG3in/LConn2
  74-75 11/RConn1 -- 75/LConn1
  47 Y I/LConn2 -- 47-48 4/RConn2 -- 47/LConn2
  73/LConn1 -- 72-73 11/RConn1 -- 73 Y PQ/LConn1
  70-71 1/RConn1 -- 71/LConn1
  28-29 2/RConn3 -- 29/LConn3
  70 Y PQ/LConn1 -- 70-71 1/LConn1 -- 70/RConn1
  17 Y PQ/LConn1 -- 17/RConn1
  21/RConn2 -- 21-23 2/LConn2 -- 21-22 10/LConn1
  69-70 9/RConn1 -- 70/LConn1
  54-55 1/LConn3 -- 54/RConn3
  35/LConn1 -- 135-35 4/RConn1 -- 35-40 1/LConn1
  60/LConn2 -- 60-62 12/LConn2 -- 60-61 5/LConn2 -- 60-1/LConn2
  12 Y PQ/LConn1 -- 12/RConn1
  1-7 1/RConn2 -- 7/LConn2
  67-72 3/LConn2 -- 67/LConn2
  87-89 6/RConn2 -- 89/LConn2
  86-87 6/RConn2 -- 87/LConn2
  8-13 1/LConn3 -- 8/RConn3
  8-13 1/RConn1 -- 13/LConn1
  8-13 1/LConn2 -- 8/RConn2
  8/LConn1 -- 7-8 1/RConn1 -- 8-9 9/LConn1
  93-95 6/LConn2 -- 93/RConn2
  89/RConn2 -- 89-91 6/LConn2 -- 89-90 10/LConn1
  16/RConn1 -- 16 Y PQ/LConn1
  5/LConn1 -- 3-5 11/RConn1
  3-4 11/RConn1 -- 4/LConn1
  13/LConn3 -- 8-13 1/RConn3 -- 13-34 11/LConn1
  9/RConn1 -- 9-14 9/LConn1 -- 9 Y PQ/LConn1
  13/RConn1 -- 13-18 2/LConn1 -- 13-152/LConn1
  13/RConn3 -- 13-18 2/LConn3 -- 13-152/LConn3
  13-18 2/RConn2 -- 18/LConn2
  13-18 2/RConn1 -- 18/LConn1
  13-18 2/RConn3 -- 18/LConn3
  10 Y I/LConn1 -- 10/RConn1
  14/RConn1 -- 14-11 9/LConn1 -- 14-10 9/RConn1
  8-13 1/LConn1 -- 8/RConn1
  7/LConn1 -- 1-7 1/RConn1 -- 7 Y PQ/LConn1
  1-7 1/RConn3 -- 7/LConn3
  47-49 4/LConn1 -- 47/RConn1
  15/RConn1 -- 15-16 11/LConn1 -- 15-17 11/LConn1
  42-44 1/LConn1 -- 42/RConn1
  14-11 9/RConn1 -- 11/LConn1
  13-34 11/RConn1 -- 34/LConn1
  52-53 1/RConn3 -- 53/LConn3
  1-3 11/RConn1 -- 3/LConn1
  57/RConn2 -- 57-58 10/RConn1 -- 54-57 3/RConn2
  18-21 2/RConn3 -- 21/LConn3
  73-74 11/LConn1 -- 73/RConn1
  74-75 11/LConn1 -- 74/RConn1
  53-54 1/LConn1 -- 53/RConn1
  52-53 1/LConn2 -- 52/RConn2
  53-54 1/LConn3 -- 53/RConn3
  52-53 1/RConn2 -- 53/LConn2
  18-21 2/RConn2 -- 21/LConn2
  35 D PQ/LConn1 -- Load Flow Bus2/RConn1 -- 35-36 8/LConn1
  53 Y PQ/LConn1 -- 52-53 1/RConn1 -- 53/LConn1
  52-53 1/LConn3 -- 52/RConn3
  53-54 1/LConn2 -- 53/RConn2
  35/LConn2 -- 135-35 4/RConn2 -- 35-40 1/LConn2
  65-66 12/LConn2 -- 65/RConn2
  62-63 12/RConn3 -- 63/LConn3
  58 Y I/LConn1 -- 58-59 10/RConn1 -- 58/RConn1
  6/LConn1 -- 5-6 11/RConn1
  19-20 9/LConn1 -- 19/RConn1
  57-60 3/RConn1 -- 60/RConn1
  5/RConn1 -- 5-6 11/LConn1 -- 5 Y I/LConn1
  63-64 12/LConn1 -- 63/RConn1
  63-64 12/LConn2 -- 63/RConn2
  69 Y PQ/LConn1 -- 69/RConn1 -- 69-70 9/LConn1
  60-62 12/RConn1 -- 62/LConn1
  24 Y PQ/LConn1 -- 24/RConn1
  28-29 2/RConn2 -- 29/LConn2
  54-57 3/RConn1 -- 57/RConn1
  29-30 2/LConn1 -- 29/RConn1
  60/LConn3 -- 60-62 12/LConn3 -- 60-61 5/LConn3 -- 60-1/LConn3
  2 Y PQ/LConn1 -- 2/RConn1
  97-98 3/RConn2 -- 98/LConn2
  63-64 12/LConn3 -- 63/RConn3
  8-13 1/RConn2 -- 13/LConn2
  8/LConn2 -- 7-8 1/RConn2 -- 8-12 10/LConn1
  42/RConn2 -- 42-43 10/LConn1 -- 42-44 1/LConn2
  3/RConn1 -- 3-4 11/LConn1 -- 3-5 11/LConn1
  1/LConn2 -- 1-2 10/LConn1 -- 149-1 1/RConn2
  13/RConn2 -- 13-18 2/LConn2 -- 13-152/LConn2
  8-9 9/RConn1 -- 9/LConn1
  7-8 1/RConn3 -- 8/LConn3
  76/LConn1 -- 76-77 6/LConn1 -- 72-76 3/RConn1
  52-53 1/LConn1 -- 52/RConn1
  40/RConn3 -- 40-41 11/LConn1 -- 40-42 1/LConn3
  28-29 2/LConn3 -- 28/RConn3
  38 Y I/LConn1 -- 38-39 10/LConn1 -- 38/RConn1
  54-57 3/RConn3 -- 57/RConn3
  40-41 11/RConn1 -- 41/LConn1
  57-60 3/RConn2 -- 60/RConn2
  60 Y PQ/LConn1 -- 60/LConn1 -- 60-62 12/LConn1 -- 60-61 5/LConn1 -- 60-1/LConn1
  18-21 2/RConn1 -- 21/LConn1
  23/RConn3 -- 23-25 2/LConn3 -- 23-24 11/LConn1
  29-30 2/LConn2 -- 29/RConn2
  29-30 2/RConn1 -- "30 "/LConn1
  44/RConn1 -- 44-45 9/LConn1 -- 44-47 1/LConn1
  60-62 12/RConn2 -- 62/LConn2
  63-64 12/RConn1 -- 64/LConn1
  67-97 3/RConn2 -- 97/LConn2
  29-30 2/LConn3 -- 29/RConn3
  67/RConn2 -- 67-97 3/LConn2 -- RG4out/RConn2
  29/LConn1 -- 28-29 2/RConn1 -- 29 Y Z/LConn1
  47 Y I/LConn3 -- 47-48 4/RConn3 -- 47/LConn3
  76/LConn2 -- 76-77 6/LConn2 -- 72-76 3/RConn2
  76/LConn3 -- 76-77 6/LConn3 -- 72-76 3/RConn3
  57-60 3/RConn3 -- 60/RConn3
  28-29 2/LConn1 -- 28/RConn1
  28-29 2/LConn2 -- 28/RConn2
  62-63 12/RConn2 -- 63/LConn2
  54/LConn3 -- 54-57 3/LConn3 -- 53-54 1/RConn3
  22 Y Z/LConn1 -- 22/RConn1
  49-50 4/LConn3 -- 49/RConn3
  21-23 2/RConn2 -- 23/LConn2
  67-97 3/LConn1 -- RG4out/RConn1 -- 67-68 9/LConn1 -- 67/RConn1
  62-63 12/LConn3 -- 62/RConn3
  45-46 9/LConn1 -- 45/RConn1
  49 Y PQ/LConn1 -- 47-49 4/RConn1 -- 49/LConn1
  30 Y PQ/LConn1 -- 29-30 2/RConn3 -- "30 "/LConn3
  54-55 1/LConn1 -- 54/RConn1
  21-23 2/RConn3 -- 23/LConn3
  30-250 2/RConn1 -- 250/LConn1
  26-31 1/RConn1 -- 31/LConn1
  40-42 1/LConn1 -- 40/RConn1
  23-25 2/LConn2 -- 23/RConn2
  65-66 12/LConn3 -- 65/RConn3
  66 Y PQ/LConn1 -- Load Flow Bus128/LConn3 -- 66/RConn3
  67-72 3/LConn1 -- 67/LConn1
  68-69 9/RConn1 -- 69/LConn1
  29-30 2/RConn2 -- "30 "/LConn2
  62 Y Z/LConn1 -- 60-62 12/RConn3 -- 62/LConn3
  21-23 2/RConn1 -- 23/LConn1
  19 Y PQ/LConn1 -- 18-19 9/RConn1 -- 19/LConn1
  58-59 10/LConn1 -- 59/LConn1
  67-72 3/RConn1 -- 72/LConn1
  23-25 2/RConn2 -- 25/LConn2
  48/RConn2 -- 44-47 1/RConn2 -- 47-48 4/LConn2
  67-68 9/RConn1 -- 68/LConn1
  49-50 4/LConn1 -- 49/RConn1
  65-66 12/LConn1 -- 65/RConn1
  48/RConn1 -- 44-47 1/RConn1 -- 47-48 4/LConn1
  63 Y PQ/LConn1 -- 62-63 12/RConn1 -- 63/LConn1
  25-28 2/RConn3 -- 28/LConn3
  21-23 2/LConn3 -- 21/RConn3
  62-63 12/LConn2 -- 62/RConn2
  46/RConn1 -- 46 Y PQ/LConn1
  47 Y I/LConn1 -- 47-48 4/RConn1 -- 47/LConn1
  67/LConn3 -- 67-72 3/LConn3 -- 72-73 11/LConn1
  62-63 12/LConn1 -- 62/RConn1
  64 Y I/LConn1 -- 63-64 12/RConn2 -- 64/LConn2
  48/RConn3 -- 44-47 1/RConn3 -- 47-48 4/LConn3
  25-28 2/RConn2 -- 28/LConn2
  28 Y I/LConn1 -- 25-28 2/RConn1 -- 28/LConn1
  31 Y PQ/LConn1 -- 31-32 1/LConn1 -- 31/RConn1
  30-250 2/RConn2 -- 250/LConn2
  34/RConn1 -- 34-15 11/LConn1 -- 34 Y Z/LConn1
  35/LConn3 -- 135-35 4/RConn3 -- 35-40 1/LConn3
  36-37 9/RConn1 -- 37/LConn1
  36-38 10/LConn1 -- Load Flow Bus55/RConn2
  36-38 10/RConn1 -- 38/LConn1
  67-97 3/RConn1 -- 97/LConn1
  30-250 2/RConn3 -- 250/LConn3
  32 Y PQ/LConn1 -- 32/RConn1
  49-50 4/RConn1 -- 50/LConn1
  40-42 1/RConn3 -- 42/LConn3
  40-42 1/RConn2 -- 42/LConn2
  42-44 1/RConn3 -- 44/LConn3
  42-44 1/RConn2 -- 44/LConn2
  68 Y PQ/LConn1 -- 68-69 9/LConn1 -- 68/RConn1
  42-44 1/RConn1 -- 44/LConn1
  42-43 10/RConn1 -- 43/LConn1
  42 Y PQ/LConn1 -- 40-42 1/RConn1 -- 42/LConn1
  47-49 4/LConn3 -- 47/RConn3
  42-44 1/LConn3 -- 42/RConn3
  39/RConn1 -- 39 Y PQ/LConn1
  65 D Z/LConn2 -- 64-65 12/RConn2 -- 65/LConn2
  40-42 1/LConn2 -- 40/RConn2
  49-50 4/RConn2 -- 50/LConn2
  50 Y PQ/LConn1 -- 49-50 4/RConn3 -- 50/LConn3
  67-97 3/RConn3 -- 97/LConn3
  45 Y I/LConn1 -- 45/LConn1 -- 44-45 9/RConn1
  23-25 2/LConn1 -- 23/RConn1
  67/RConn3 -- 67-97 3/LConn3 -- RG4out/RConn3
  19-20 9/RConn1 -- 20/LConn1
  35 D PQ/RConn1 -- 35-36 8/LConn2 -- Load Flow Bus2/RConn2
  67-72 3/RConn2 -- 72/LConn2
  54-55 1/LConn2 -- 54/RConn2
  25/LConn1 -- 23-25 2/RConn1 -- RG3in/LConn1
  49 Y PQ/LConn3 -- 47-49 4/RConn3 -- 49/LConn3
  49 Y PQ/LConn2 -- 47-49 4/RConn2 -- 49/LConn2
  49-50 4/LConn2 -- 49/RConn2
  47-49 4/LConn2 -- 47/RConn2
  63-64 12/RConn3 -- 64/LConn3
  36/LConn1 -- 36-37 9/LConn1 -- 35-36 8/RConn1
  54/LConn2 -- 54-57 3/LConn2 -- 53-54 1/RConn2
  Ground7/LConn1 -- 10 Y I/RConn1
  250-251/RConn2 -- Load Flow Bus10/LConn2
  Ground5/LConn1 -- 7 Y PQ/RConn1
  Ground4/LConn1 -- 5 Y I/RConn1
  Ground1/LConn1 -- 2 Y PQ/RConn1
  76-86 3/RConn1 -- 86/LConn1
  60-61 5/RConn3 -- 61/LConn3
  Ground6/LConn1 -- 9 Y PQ/RConn1
  94/LConn1 -- 59-94/RConn1
  450-451/RConn2 -- Load Flow Bus107/LConn2
  Ground8/LConn1 -- 11 Y Z/RConn1
  Ground3/LConn1 -- 6 Y Z/RConn1
  77-78 6/RConn2 -- 78/LConn2
  77-78 6/RConn1 -- 78/LConn1
  Load Flow Bus78/LConn1 -- Three-Phase Breaker1/RConn1
  76 DI/LConn3 -- 76-86 3/LConn3 -- 76/RConn3
  76-86 3/RConn2 -- 86/LConn2
  60-61 5/RConn2 -- 61/LConn2
  Load Flow Bus78/LConn3 -- Three-Phase Breaker1/RConn3
  Ground/LConn1 -- 1 Y PQ/RConn1
  Load Flow Bus78/LConn2 -- Three-Phase Breaker1/RConn2
  Ground9/LConn1 -- 12 Y PQ/RConn1
  Ground10/LConn1 -- 16 Y PQ/RConn1
  Ground11/LConn1 -- 17 Y PQ/RConn1
  Ground12/LConn1 -- 19 Y PQ/RConn1
  Ground13/LConn1 -- 20 Y I/RConn1
  Ground14/LConn1 -- 22 Y Z/RConn1
  Ground15/LConn1 -- 24 Y PQ/RConn1
  Ground16/LConn1 -- 28 Y I/RConn1
  Ground17/LConn1 -- 29 Y Z/RConn1
  Ground18/LConn1 -- 30 Y PQ/RConn1
  Ground19/LConn1 -- 31 Y PQ/RConn1
  Ground20/LConn1 -- 32 Y PQ/RConn1
  Ground21/LConn1 -- 33 Y I/RConn1
  Ground22/LConn1 -- 34 Y Z/RConn1
  Ground23/LConn1 -- 37 Y Z/RConn1
  Ground24/LConn1 -- 38 Y I/RConn1
  Ground25/LConn1 -- 39 Y PQ/RConn1
  Ground26/LConn1 -- 41 Y PQ/RConn1
  Ground27/LConn1 -- 42 Y PQ/RConn1
  Ground28/LConn1 -- 43 Y Z/RConn1
  Ground29/LConn1 -- 45 Y I/RConn1
  Ground30/LConn1 -- 46 Y PQ/RConn1
  Ground31/LConn1 -- 50 Y PQ/RConn1
  Ground32/LConn1 -- 51 Y PQ/RConn1
  Ground33/LConn1 -- 52 Y PQ/RConn1
  Ground34/LConn1 -- 53 Y PQ/RConn1
  Ground35/LConn1 -- 55 Y Z/RConn1
  Ground36/LConn1 -- 56 Y PQ/RConn1
  Ground37/LConn1 -- 58 Y I/RConn1
  Ground38/LConn1 -- 59 Y PQ/RConn1
  Ground39/LConn1 -- 60 Y PQ/RConn1
  Ground40/LConn1 -- 62 Y Z/RConn1
  Ground41/LConn1 -- 63 Y PQ/RConn1
  Ground42/LConn1 -- 64 Y I/RConn1
  Ground43/LConn1 -- 66 Y PQ/RConn1
  Ground44/LConn1 -- 68 Y PQ/RConn1
  Ground45/LConn1 -- 69 Y PQ/RConn1
  Ground46/LConn1 -- 70 Y PQ/RConn1
  Ground47/LConn1 -- 71 Y PQ/RConn1
  Ground48/LConn1 -- 73 Y PQ/RConn1
  Ground49/LConn1 -- 74 Y Z/RConn1
  Ground50/LConn1 -- 75 Y PQ/RConn1
  Ground51/LConn1 -- 77 Y PQ/RConn1
  Ground52/LConn1 -- 79 Y Z/RConn1
  Ground53/LConn1 -- 80 Y PQ/RConn1
  Ground54/LConn1 -- 82 Y PQ/RConn1
  Ground55/LConn1 -- 83 Y PQ/RConn1
  Ground56/LConn1 -- 84 Y PQ/RConn1
  Ground57/LConn1 -- 85 Y PQ/RConn1
  Ground58/LConn1 -- 86 Y PQ/RConn1
  Ground59/LConn1 -- 87 Y PQ/RConn1
  Ground60/LConn1 -- 88 Y PQ/RConn1
  Ground61/LConn1 -- 90 Y I/RConn1
  Ground62/LConn1 -- 92 Y PQ/RConn1
  Ground63/LConn1 -- 94 Y PQ/RConn1
  Ground64/LConn1 -- 95 Y PQ/RConn1
  Ground65/LConn1 -- 96 Y PQ/RConn1
  Ground66/LConn1 -- 98 Y PQ/RConn1
  Ground67/LConn1 -- 99 Y PQ/RConn1
  Ground68/LConn1 -- 100 Y Z/RConn1
  Ground69/LConn1 -- 102 Y Z/RConn1
  Ground70/LConn1 -- 103 Y PQ/RConn1
  Ground71/LConn1 -- 104 Y PQ/RConn1
  Ground72/LConn1 -- 106 Y PQ/RConn1
  Ground73/LConn1 -- 107 Y PQ/RConn1
  Ground74/LConn1 -- 109 Y PQ/RConn1
  Ground75/LConn1 -- 111 Y PQ/RConn1
  Ground76/LConn1 -- 112 Y I/RConn1
  Ground77/LConn1 -- 113 Y Z/RConn1
  Ground78/LConn1 -- 114 Y PQ/RConn1
  83/RConn1 -- 83 Y CAP/LConn1
  83/RConn2 -- 83 Y CAP/LConn2
  83/RConn3 -- 83 Y CAP/LConn3
  Ground79/LConn1 -- 88 Y CAP/RConn1
  Ground80/LConn1 -- 90 Y CAP/RConn1
  Ground81/LConn1 -- 92 Y CAP/RConn1
  149-1 1/RConn3 -- 1/LConn3
  149-1 1/LConn3 -- 149/RConn3
  197-101 3/RConn2 -- 101/LConn2
  76 DI/LConn2 -- 76-86 3/LConn2 -- 76/RConn2
  77-78 6/RConn3 -- 78/LConn3
  100-450 3/LConn1 -- 100/RConn1
  78/RConn1 -- 78-80 6/LConn1 -- 78-79 6/LConn1
  99-100 3/RConn1 -- 100/LConn1
  78/RConn3 -- 78-80 6/LConn3 -- 78-79 6/LConn3
  99-100 3/RConn2 -- 100/LConn2
  99-100 3/RConn3 -- 100/LConn3
  99 Y PQ/LConn1 -- 99-100 3/LConn2 -- 99/RConn2
  76-77 6/RConn3 -- 77/LConn3
  77/LConn2 -- 76-77 6/RConn2 -- 77 Y PQ/LConn1
  76-77 6/RConn1 -- 77/LConn1
  149-1 1/LConn2 -- 149/RConn2
  149-1 1/RConn1 -- 1/LConn1
  197-101 3/RConn3 -- 101/LConn3
  149-1 1/LConn1 -- 149/RConn1
  135-35 4/LConn3 -- 135/RConn3
  52 Y PQ/LConn1 -- 152-52 1/RConn1 -- 52/LConn1
  135-35 4/LConn2 -- 135/RConn2
  135-35 4/LConn1 -- 135/RConn1
  152-52 1/RConn2 -- 52/LConn2
  113-114 9/RConn1 -- 114/LConn1
  113 Y Z/LConn1 -- 113-114 9/LConn1 -- 113/RConn1
  152-52 1/RConn3 -- 52/LConn3
  112-113 9/RConn1 -- 113/LConn1
  152-52 1/LConn1 -- 152/RConn1
  112 Y I/LConn1 -- 112/RConn1 -- 112-113 9/LConn1
  110-112 9/RConn1 -- 112/LConn1
  152-52 1/LConn2 -- 152/RConn2
  110-111 9/RConn1 -- 111/LConn1
  152-52 1/LConn3 -- 152/RConn3
  110/LConn1 -- 110-111 9/LConn1 -- 109-110 9/RConn1
  109/RConn1 -- 109-110 9/LConn1 -- 109 Y PQ/LConn1
  450-451/RConn3 -- Load Flow Bus107/LConn3
  250-251/RConn3 -- Load Flow Bus10/LConn3
  300/LConn3 -- 108-300 3/RConn3 -- 151-1/RConn3
  300/LConn2 -- 108-300 3/RConn2 -- 151-1/RConn2
  300/LConn1 -- 108-300 3/RConn1 -- 151-1/RConn1
  108-109 9/RConn1 -- 109/LConn1
  107 Y PQ/LConn1 -- 107/RConn1
  106 Y PQ/LConn1 -- 106-107 10/LConn1 -- 106/RConn1
  60-61 5/RConn1 -- 61/LConn1
  105/RConn2 -- 105-108 3/LConn2 -- 105-106 10/LConn1
  105-108 3/LConn3 -- 105/RConn3
  105-108 3/LConn1 -- 105/RConn1
  105-108 3/RConn3 -- 108/LConn3
  105-108 3/RConn2 -- 108/LConn2
  105-108 3/RConn1 -- 108/LConn1
  105-106 10/RConn1 -- 106/LConn1
  60-1/RConn1 -- 160/LConn1
  101-105 3/RConn2 -- 105/LConn2
  60-1/RConn2 -- 160/LConn2
  105/LConn3 -- 101-102 11/LConn1 -- 101-105 3/RConn3
  60-1/RConn3 -- 160/LConn3
  101-105 3/RConn1 -- 105/LConn1
  103 Y PQ/LConn1 -- 103-104 11/LConn1 -- 103/RConn1
  104 Y PQ/LConn1 -- 104/RConn1
  197-101 3/LConn2 -- 197/RConn2
  102-103 11/RConn1 -- 103/LConn1
  102/RConn1 -- 102-103 11/LConn1 -- 102 Y Z/LConn1
  197-101 3/LConn3 -- 197/RConn3
  101-102 11/RConn1 -- 102/LConn1
  197-101 3/RConn1 -- 101/LConn1
  100 Y Z/LConn1 -- 100-450 3/LConn3 -- 100/RConn3
  100-450 3/LConn2 -- 100/RConn2
  92 Y PQ/LConn1 -- 92/RConn1 -- 92 Y CAP/LConn1
  91/RConn3 -- 91-93 6/LConn3 -- 91-92 11/LConn1
  Ground2/LConn1 -- 4Y PQ/RConn1
  89-91 6/RConn3 -- 91/LConn3
  89-91 6/RConn2 -- 91/LConn2
  89-91 6/RConn1 -- 91/LConn1
  93/RConn1 -- 93-95 6/LConn1 -- 93-94 9/LConn1
  89-91 6/LConn3 -- 89/RConn3
  89-91 6/LConn1 -- 89/RConn1
  90 Y CAP/LConn1 -- 90/RConn1 -- 90 Y I/LConn1
  87-89 6/RConn3 -- 89/LConn3
  87-89 6/RConn1 -- 89/LConn1
  87/RConn1 -- 87-89 6/LConn1 -- 87-88 9/LConn1
  450-451/RConn1 -- Load Flow Bus107/LConn1
  88 Y CAP/LConn1 -- 88/RConn1 -- 88 Y PQ/LConn1
  95-96 10/LConn1 -- Load Flow Bus77/LConn2
  86-87 6/RConn3 -- 87/LConn3
  86-87 6/RConn1 -- 87/LConn1
  93-95 6/LConn3 -- 93/RConn3
  86-87 6/LConn3 -- 86/RConn3
  86 Y PQ/LConn1 -- 86-87 6/LConn2 -- 86/RConn2
  97-98 3/RConn1 -- 98/LConn1
  150/RConn2 -- 150-1/LConn2
  86-87 6/LConn1 -- 86/RConn1
  95-96 10/RConn1 -- 96/LConn1
  83 Y PQ/LConn1 -- 82-83 6/RConn3 -- 83/LConn3
  97-98 3/RConn3 -- 98/LConn3
  82-83 6/RConn2 -- 83/LConn2
  82-83 6/RConn1 -- 83/LConn1
  82-83 6/LConn3 -- 82/RConn3
  82-83 6/LConn2 -- 82/RConn2
  82 Y PQ/LConn1 -- 82-83 6/LConn1 -- 82/RConn1
  84-85 11/RConn1 -- 85/LConn1
  84-85 11/LConn1 -- 84/RConn1
  98-99 3/RConn1 -- 99/LConn1
  84 Y PQ/LConn1 -- 81-84 11/RConn1 -- 84/LConn1
  250-251/RConn1 -- Load Flow Bus10/LConn1
  98-99 3/RConn2 -- 99/LConn2
  81-82 6/RConn3 -- 82/LConn3
  81-82 6/RConn2 -- 82/LConn2
  98-99 3/RConn3 -- 99/LConn3
  81-82 6/RConn1 -- 82/LConn1
  81/RConn3 -- 81-84 11/LConn1 -- 81-82 6/LConn3
  99-100 3/LConn1 -- 99/RConn1
  76 DI/LConn1 -- 76-86 3/LConn1 -- 76/RConn1
  91-93 6/LConn1 -- 91/RConn1
  80-81 6/RConn3 -- 81/LConn3
  91-93 6/LConn2 -- 91/RConn2
  80-81 6/RConn2 -- 81/LConn2
  80-81 6/RConn1 -- 81/LConn1
  80-81 6/LConn3 -- 80/RConn3
  94 Y PQ/LConn1 -- 93-94 9/RConn1 -- 94/RConn1
  80 Y PQ/LConn1 -- 80-81 6/LConn2 -- 80/RConn2
  80-81 6/LConn1 -- 80/RConn1
  78-80 6/RConn3 -- 80/LConn3
  78-80 6/RConn2 -- 80/LConn2
  97-1/LConn1 -- 97-98 3/LConn1 -- 97/RConn1
  97/RConn3 -- 97-98 3/LConn3 -- 97-1/LConn3
  97-1/LConn2 -- 97-98 3/LConn2 -- 97/RConn2
  197-101 3/LConn1 -- 197/RConn1
  99-100 3/LConn3 -- 99/RConn3
  76-86 3/RConn3 -- 86/LConn3
  79 Y Z/LConn1 -- Load Flow Bus117/LConn1 -- 79/RConn1
  78/RConn2 -- 78-80 6/LConn2 -- 78-79 6/LConn2
  78-80 6/RConn1 -- 80/LConn1
  Regulator 4/LConn1 -- RG4in/RConn1
  RG4in/RConn2 -- Regulator 4/LConn2
  RG4in/RConn3 -- Regulator 4/LConn3
  Regulator 4/RConn1 -- RG4out/LConn1
  Regulator 4/RConn2 -- RG4out/LConn2
  Regulator 4/RConn3 -- RG4out/LConn3
  Regulator 2/LConn1 -- RG2in/RConn1
  Regulator 2/RConn1 -- RG2out/LConn1
  26/RConn1 -- 26-27 7/LConn2
  26-27 7/RConn2 -- 27/LConn1
  27/LConn2 -- 26-27 7/RConn1
  26/RConn2 -- 26-27 7/LConn1
  26/LConn1 -- 25-26 1/RConn2
  25-26 1/LConn2 -- RG3out/RConn1
  25-26 1/LConn1 -- RG3out/RConn2
  Regulator 3/RConn1 -- RG3out/LConn1
  Regulator 3/RConn2 -- RG3out/LConn2
  Regulator 3/LConn1 -- RG3in/RConn1
  Regulator 3/LConn2 -- RG3in/RConn2
